simulink model "closedloop_linear_2015b"  (R2015b)
settings: Solver=ode45  StartTime=0.0  StopTime=2000  RelTol=1e-3
values from neighbouring files (symbols this model uses):
  model = block.DialogPrm(2).Data    [sfun_mpc.m]
  mpc = mpc_design(model,rho,60,20,model.u_lb,model.u_ub,'delta')    [init.m]    (also in sfun_mpc.m = block.DialogPrm(1).Data)
settings Model: Creator=schauer  LastModifiedBy=schauer
settings DataIOCC: SaveFormat=Array
settings DebuggingCC: SolverPrmCheckMsg=warning  AllowSymbolicDim=on
settings HardwareCC: ProdBitPerPointer=32  ProdLargestAtomicFloat=None  ProdIntDivRoundTo=Undefined  ProdEndianess=Unspecified  ProdWordSize=32  ProdHWDeviceType=32-bit Generic
settings GRTTargetCC: GeneratePreprocessorConditionals=Disable all
settings ConfigComp: CovModelRefEnable=Off  CovSFcnEnable=off

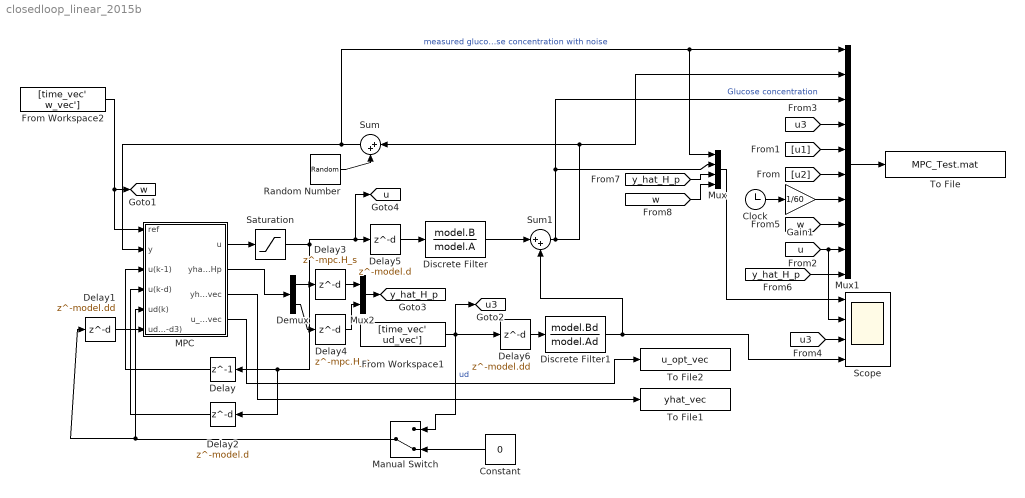
== system closedloop_linear_2015b ==
  Clock : Clock
  Constant : Constant  Value=0
  Delay : Delay  DelayLength=1  InitialCondition=0  SampleTime=model.Ts
  Delay1 : Delay  DelayLength=model.dd  InitialCondition=0  SampleTime=model.Ts
  Delay2 : Delay  DelayLength=model.d  InitialCondition=0  SampleTime=model.Ts
  Delay3 : Delay  DelayLength=mpc.H_s  InitialCondition=0  SampleTime=model.Ts
  Delay4 : Delay  DelayLength=mpc.H_p  InitialCondition=0  SampleTime=model.Ts
  Delay5 : Delay  DelayLength=model.d  InitialCondition=0  SampleTime=model.Ts
  Delay6 : Delay  DelayLength=model.dd  InitialCondition=0  SampleTime=model.Ts
  Demux : Demux  Outputs=2
  Discrete Filter : DiscreteFilter  Numerator=model.B  Denominator=model.A  InitialStates=[0 0]  InitialDenominatorStates=[60 60 60 60]  FilterStructure=Direct form I
  Discrete Filter1 : DiscreteFilter  Numerator=model.Bd  Denominator=model.Ad
  From Workspace1 : FromWorkspace  VariableName=[time_vec' ud_vec']  SampleTime=0  Interpolate=off  OutputAfterFinalValue=Setting to zero
  From Workspace2 : FromWorkspace  VariableName=[time_vec' w_vec']  SampleTime=0  Interpolate=off  OutputAfterFinalValue=Setting to zero
  Gain1 : Gain  Gain=1/60  SampleTime=model.Ts
  MPC : Subsystem
  Manual Switch : ManualSwitch  CurrentSetting=0
  Mux : Mux
  Mux1 : Mux  Inputs=10
  Mux2 : Mux  Inputs=2
  Random Number : RandomNumber  Variance=10  SampleTime=model.Ts
  Saturation : Saturate  UpperLimit=800  LowerLimit=-1000
  Scope : Scope  NumInputPorts=4
  Sum : Sum  Inputs=|++
  Sum1 : Sum  Inputs=|++
  To File : ToFile  Filename=MPC_Test.mat  MatrixName=MPC_data  SampleTime=model.Ts
  To File1 : ToFile  Filename=yhat_vec  MatrixName=yhat_vec  SampleTime=model.Ts
  To File2 : ToFile  Filename=u_opt_vec  MatrixName=u_opt_vec  SampleTime=model.Ts
  tag scope: u3=global, u=global, w=global, y_hat_H_p=global
  wires:
  From Workspace1/1 -> Manual Switch/1, [u3], Delay6/1  "ud"
  Manual Switch/1 -> MPC/5(ud(k)), Delay1/1
  MPC/1(u) -> Saturation/1
  From Workspace2/1 -> MPC/1(ref), [w]
  Delay1/1 -> MPC/6(ud(k-d3))
  Sum1/1 -> Mux1/2, Sum/1, Mux1/3, Mux/2  "Glucose concentration"
  Delay/1 -> MPC/3(u(k-1))
  Delay2/1 -> MPC/4(u(k-d))
  Random Number/1 -> Sum/2
  Sum/1 -> MPC/2(y), Mux/1, Mux1/1  "measured glucose concentration with noise"
  Mux/1 -> Scope/1
  Mux1/1 -> To File/1
  [u1] -> Mux1/5
  [u2] -> Mux1/6
  Clock/1 -> Gain1/1
  Gain1/1 -> Mux1/7
  MPC/2("yhat_Hp ") -> Demux/1
  [u] -> Scope/2, Mux1/9
  [u3] -> Mux1/4
  [u3] -> Scope/3
  [w] -> Mux1/8
  [y_hat_H_p] -> Mux1/10
  Mux2/1 -> [y_hat_H_p]
  Constant/1 -> Manual Switch/2
  Demux/1 -> Delay3/1
  Delay3/1 -> Mux2/1
  Demux/2 -> Delay4/1
  Delay4/1 -> Mux2/2
  Discrete Filter1/1 -> Sum1/2, Scope/4
  Discrete Filter/1 -> Sum1/1
  Delay6/1 -> Discrete Filter1/1
  Delay5/1 -> Discrete Filter/1
  MPC/3("yhat_vec ") -> To File1/1
  MPC/4(u_opt_vec) -> To File2/1
  Saturation/1 -> [u], Delay5/1, Delay2/1, Delay/1
  [w] -> Mux/4
  [y_hat_H_p] -> Mux/3

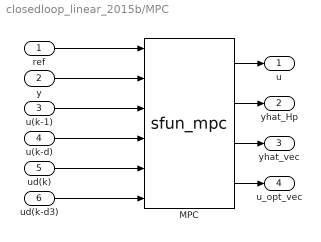
== system closedloop_linear_2015b/MPC ==
  ref : Inport
  y : Inport  Port=2
  u(k-1) : Inport  Port=3
  u(k-d) : Inport  Port=4
  ud(k) : Inport  Port=5
  ud(k-d3) : Inport  Port=6
  MPC : M-S-Function  FunctionName=sfun_mpc  Parameters=mpc,model
  u : Outport
  "yhat_Hp " : Outport  Port=2
  "yhat_vec " : Outport  Port=3
  u_opt_vec : Outport  Port=4
  wires:
  MPC/1 -> u/1
  ref/1 -> MPC/1
  y/1 -> MPC/2
  u(k-1)/1 -> MPC/3
  u(k-d)/1 -> MPC/4
  ud(k)/1 -> MPC/5
  ud(k-d3)/1 -> MPC/6
  MPC/2 -> "yhat_Hp "/1
  MPC/3 -> "yhat_vec "/1
  MPC/4 -> u_opt_vec/1
